simulink model "V2G_sim"  (R2021a)
settings: Solver=VariableStepAuto  StartTime=0  StopTime=tmax  FixedStep=sample_time  RelTol=1e-3  EnableMultiTasking=on
values from neighbouring files (symbols this model uses):
  Cap_car3_SC = 165    [V2G.m]
  grid_voltage = 230*sqrt(3)    [V2G.m]
  num_car1 = randi([1,50])    [V2G.m]
  num_car2 = randi([1,50])    [V2G.m]
  num_car3 = randi([1,50])    [V2G.m]
  pun = 40    [V2G.m]
  Qacc_MEAN = mean(Qacc_TOT, 1)    [V2G.m]
  sample_time = 0.0005    [V2G.m]
  V_car3_SC = 48    [V2G.m]
undefined symbols (not defined in the file or in its folder): Ion, Lithium
libraries: spsBreakerLib x8, spsCurrentMeasurementLib x8, spsVoltageMeasurementLib x8, spsMosfetLib x8, spsControlledCurrentSourceLib x4, spsSeriesRLCBranchLib x4, spsBatteryLib x3, simulink x2, spsSupercapacitorLib x1, spspowerguiLib x1
Description:
  | Copyright 2008-2016 The MathWorks, Inc.
settings Model: SimulationMode=accelerator  Creator=MathWorks  LastModifiedBy=rod
settings SolverCC: AlgebraicLoopSolver=TrustRegion
settings DataIOCC: FinalStateName=OperationPoint  InitialState=OperationPoint  LimitDataPoints=on  LoadInitialState=on  SaveFinalState=on  SaveOperatingPoint=on  SaveFormat=Array  SignalLoggingSaveFormat=ModelDataLogs  ReturnWorkspaceOutputs=off
settings OptimizationCC: BlockReduction=off  DefaultParameterBehavior=Inlined  BufferReuse=off  ExpressionDepthLimit=2147483647  EfficientMapNaN2IntZero=off  LifeSpan=inf
settings DebuggingCC: UnderspecifiedInitializationDetection=Classic  MergeDetectMultiDrivingBlocksExec=none  SolverPrmCheckMsg=warning  FcnCallInpInsideContextMsg=warning  UnconnectedInputMsg=none  UnconnectedOutputMsg=none  UnconnectedLineMsg=none  AllowSymbolicDim=off  StateNameClashWarn=warning  SFUnexpectedBacktrackingDiag=warning  SFNoUnconditionalDefaultTransitionDiag=warning  SFExecutionAtInitializationDiag=none  SFMachineParentedDataDiag=warning  ArithmeticOperatorsInVariantConditions=warning
settings HardwareCC: ProdBitPerPointer=32  ProdBitPerSizeT=32  ProdBitPerPtrDiffT=32  ProdLargestAtomicFloat=None  ProdIntDivRoundTo=Undefined  ProdEndianess=Unspecified  ProdWordSize=32  ProdHWDeviceType=32-bit Generic  TargetBitPerLong=64  TargetBitPerPointer=64  TargetBitPerSizeT=64  TargetBitPerPtrDiffT=64  TargetLongLongMode=on  TargetIntDivRoundTo=Zero  TargetEndianess=LittleEndian  TargetWordSize=64  TargetHWDeviceType=MATLAB Host  ProdEqTarget=off
settings ModelReferenceCC: PropagateSignalLabelsOutOfModel=off
settings SFSimCC: SimUseLocalCustomCode=off  CustomCodeUndefinedFunction=UseInterfaceOnly
settings RTWCC: SystemTargetFile=accel.tlc  TemplateMakefile=accel_default_tmf  RTWVerbose=off  RTWUseLocalCustomCode=off
settings CodeAppCC: MaxIdLength=128  StateflowObjectComments=on
settings STFCustomTargetCC: MATLABClassNameForMDSCustomization=Simulink.SoftwareTarget.TargetSpecificTriggerConfigurationBase  UseToolchainInfoCompliant=off  SystemTargetFile=accel.tlc
settings ConfigComp: CovMetricSettings=dw  CovSaveCumulativeToWorkspaceVar=on  CovSaveSingleToWorkspaceVar=on  CovExternalEMLEnable=off  CovSFcnEnable=off
settings SimscapeCC: SimscapeNormalizeSystem=off

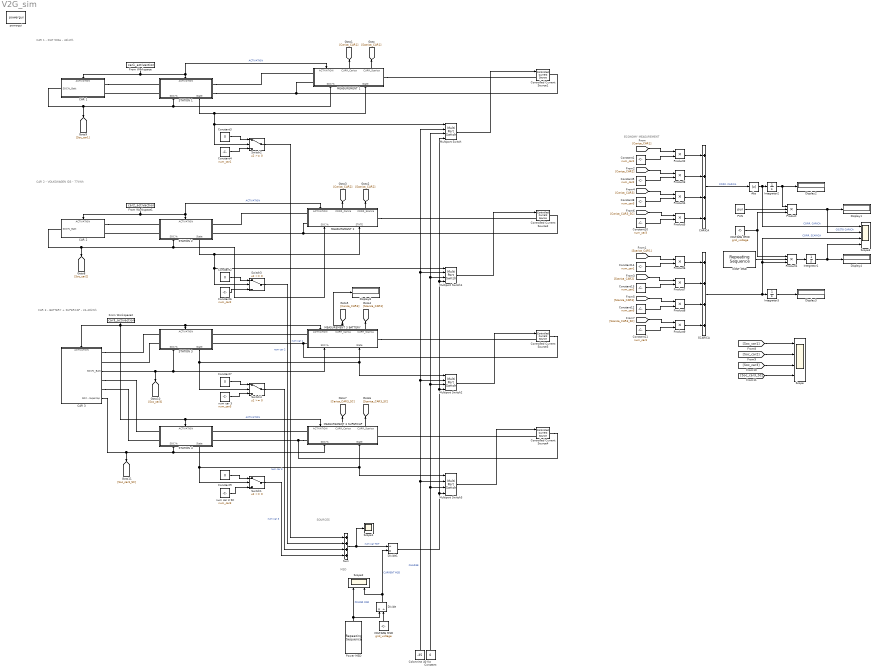
== system V2G_sim ==
  note: ECONOMY MEASUREMENT
  note: CAR 2 - VOLKSWAGEN ID3 - 77kWh
  note: SOURCES
  note: MSD
  note: CAR 1 - FIAT 500e - 42kWh
  note: CAR 3 - BATTERY + SUPERCAP - 24-40kWh
  Abs : Abs
  CAR 1 : Subsystem
      settings: PortSchema="{\"entries\":[{\"content\":{\"sides\":[{\"content\":{\"connectorIds\":[\"Out1\"]},\"type\":\"ConnectorPlacement.EquallySpacedRectSide\",\"uuid\":\"65240932-2f7c-4e6f-a11f-24cebb7f6932\"},{\"content\":{\"connectorIds\":[\"RConn1\",\"RConn2\"],\"side\":\"RIGHT\"},\"type\":\"ConnectorPlacement.EquallySpacedRectSide\",\"uuid\":\"fe08d712-a294-43ae-b558-1367f8f9eddb\"},{\"content\":{\"connectorIds\":[\"In1\"],\"side\":\"TOP\"},\"type\":\"ConnectorPlacement.EquallySpacedRectSide\",\"uuid\":\"eb8a317a-712b-4977-acdc-c1fc50b80e89\"},{\"content\":{\"connectorIds\":[],\"side\":\"BOTTOM\"},\"type\":\"ConnectorPlacement.EquallySpacedRectSide\",\"uuid\":\"4277e686-58a0-45df-b571-69968d3e8f8c\"}]},\"type\":\"ConnectorPlacement.EquallySpacedConnector\",\"uuid\":\"4b8ded93-b982-40b7-aa5b-c2f165d3142b\"}],\"packageUris\":[\"http://schema.mathworks.com/mf0/Connector/R2020b\"],\"version\":\"1.0\"}"
  CAR 2 : Subsystem
      settings: PortSchema="{\"entries\":[{\"content\":{\"sides\":[{\"content\":{\"connectorIds\":[\"Out1\"]},\"type\":\"ConnectorPlacement.EquallySpacedRectSide\",\"uuid\":\"65240932-2f7c-4e6f-a11f-24cebb7f6932\"},{\"content\":{\"connectorIds\":[\"RConn1\",\"RConn2\"],\"side\":\"RIGHT\"},\"type\":\"ConnectorPlacement.EquallySpacedRectSide\",\"uuid\":\"fe08d712-a294-43ae-b558-1367f8f9eddb\"},{\"content\":{\"connectorIds\":[\"In1\"],\"side\":\"TOP\"},\"type\":\"ConnectorPlacement.EquallySpacedRectSide\",\"uuid\":\"eb8a317a-712b-4977-acdc-c1fc50b80e89\"},{\"content\":{\"connectorIds\":[],\"side\":\"BOTTOM\"},\"type\":\"ConnectorPlacement.EquallySpacedRectSide\",\"uuid\":\"4277e686-58a0-45df-b571-69968d3e8f8c\"}]},\"type\":\"ConnectorPlacement.EquallySpacedConnector\",\"uuid\":\"4b8ded93-b982-40b7-aa5b-c2f165d3142b\"}],\"packageUris\":[\"http://schema.mathworks.com/mf0/Connector/R2020b\"],\"version\":\"1.0\"}"
  CAR 3 : Subsystem
      settings: PortSchema="{\"entries\":[{\"content\":{\"sides\":[{\"content\":{\"connectorIds\":[]},\"type\":\"ConnectorPlacement.EquallySpacedRectSide\",\"uuid\":\"65240932-2f7c-4e6f-a11f-24cebb7f6932\"},{\"content\":{\"connectorIds\":[\"RConn1\",\"RConn2\",\"Out1\",\"RConn3\",\"RConn4\",\"Out2\"],\"side\":\"RIGHT\"},\"type\":\"ConnectorPlacement.EquallySpacedRectSide\",\"uuid\":\"fe08d712-a294-43ae-b558-1367f8f9eddb\"},{\"content\":{\"connectorIds\":[\"In1\"],\"side\":\"TOP\"},\"type\":\"ConnectorPlacement.EquallySpacedRectSide\",\"uuid\":\"eb8a317a-712b-4977-acdc-c1fc50b80e89\"},{\"content\":{\"connectorIds\":[],\"side\":\"BOTTOM\"},\"type\":\"ConnectorPlacement.EquallySpacedRectSide\",\"uuid\":\"4277e686-58a0-45df-b571-69968d3e8f8c\"}]},\"type\":\"ConnectorPlacement.EquallySpacedConnector\",\"uuid\":\"4b8ded93-b982-40b7-aa5b-c2f165d3142b\"}],\"packageUris\":[\"http://schema.mathworks.com/mf0/Connector/R2020b\"],\"version\":\"1.0\"}"
  CARICA : Sum  Inputs=++++
  COST MSD : simulink/Sources/Repeating Sequence  rep_seq_t=time_var  rep_seq_y=Costo_MWh
  Colonnina 40 Kw : Constant  Value=-35
  Constant{,2..3,7,9} (5 alike) : Constant  Value=0
  Constant1 : Constant  Value=num_car1
  Constant{8,10..12} (4 alike) : Constant  Value=num_car3
  Constant13 : Constant  Value=num_car2
  Constant14 : Constant  Value=num_car1
  Constant4 : Constant  Value=num_car1
  Constant5 : Constant  Value=num_car2
  Constant6 : Constant  Value=num_car2
  Controlled Current Source{1..4} (4 alike) : spsControlledCurrentSourceLib/Controlled Current Source  Initialize=off  Source_Type=AC  Amplitude=0  Phase=0  Frequency=0  Measurements=None
  Display{1..4,8} (5 alike) : Display
  Divide : Product  Inputs=*/
  Divide1 : Product  Inputs=/*
  From Workspace : FromWorkspace  VariableName=car1_activaction  OutDataTypeStr=double  Interpolate=off  OutputAfterFinalValue=Holding final value
  From Workspace1 : FromWorkspace  VariableName=car2_activaction  OutDataTypeStr=double  Interpolate=off  OutputAfterFinalValue=Holding final value
  From Workspace2 : FromWorkspace  VariableName=car3_activaction  OutDataTypeStr=double  Interpolate=off  OutputAfterFinalValue=Holding final value
  Integrator1 : Integrator
  Integrator2 : Integrator
  Integrator3 : Integrator
  MEASUREMENT 1 : Subsystem
      settings: PortSchema="{\"entries\":[{\"content\":{\"sides\":[{\"content\":{\"connectorIds\":[\"LConn1\",\"LConn2\"]},\"type\":\"ConnectorPlacement.EquallySpacedRectSide\",\"uuid\":\"bd49ef22-917f-43a7-a189-1e95a09b9934\"},{\"content\":{\"connectorIds\":[\"RConn1\"],\"side\":\"RIGHT\"},\"type\":\"ConnectorPlacement.EquallySpacedRectSide\",\"uuid\":\"f047bc4d-f3d5-4ba6-b200-54db61941c53\"},{\"content\":{\"connectorIds\":[\"In1\",\"Out1\",\"Out2\"],\"side\":\"TOP\"},\"type\":\"ConnectorPlacement.EquallySpacedRectSide\",\"uuid\":\"9d09de71-fe9a-4093-9092-d12f300b0940\"},{\"content\":{\"connectorIds\":[\"In2\",\"In3\"],\"side\":\"BOTTOM\"},\"type\":\"ConnectorPlacement.EquallySpacedRectSide\",\"uuid\":\"f7496d22-be24-4c8d-8efb-c768b29ff46b\"}]},\"type\":\"ConnectorPlacement.EquallySpacedConnector\",\"uuid\":\"0e7a4336-45ad-4cd1-9eb0-8ed9ee74ee56\"}],\"packageUris\":[\"http://schema.mathworks.com/mf0/Connector/R2020b\"],\"version\":\"1.0\"}"
  MEASUREMENT 2 : Subsystem
      settings: PortSchema="{\"entries\":[{\"content\":{\"sides\":[{\"content\":{\"connectorIds\":[\"LConn1\",\"LConn2\"]},\"type\":\"ConnectorPlacement.EquallySpacedRectSide\",\"uuid\":\"bd49ef22-917f-43a7-a189-1e95a09b9934\"},{\"content\":{\"connectorIds\":[\"RConn1\"],\"side\":\"RIGHT\"},\"type\":\"ConnectorPlacement.EquallySpacedRectSide\",\"uuid\":\"f047bc4d-f3d5-4ba6-b200-54db61941c53\"},{\"content\":{\"connectorIds\":[\"In1\",\"Out1\",\"Out2\"],\"side\":\"TOP\"},\"type\":\"ConnectorPlacement.EquallySpacedRectSide\",\"uuid\":\"9d09de71-fe9a-4093-9092-d12f300b0940\"},{\"content\":{\"connectorIds\":[\"In2\",\"In3\"],\"side\":\"BOTTOM\"},\"type\":\"ConnectorPlacement.EquallySpacedRectSide\",\"uuid\":\"f7496d22-be24-4c8d-8efb-c768b29ff46b\"}]},\"type\":\"ConnectorPlacement.EquallySpacedConnector\",\"uuid\":\"0e7a4336-45ad-4cd1-9eb0-8ed9ee74ee56\"}],\"packageUris\":[\"http://schema.mathworks.com/mf0/Connector/R2020b\"],\"version\":\"1.0\"}"
  MEASUREMENT 3 BATTERY : Subsystem
      settings: PortSchema="{\"entries\":[{\"content\":{\"sides\":[{\"content\":{\"connectorIds\":[\"LConn1\",\"LConn2\"]},\"type\":\"ConnectorPlacement.EquallySpacedRectSide\",\"uuid\":\"bd49ef22-917f-43a7-a189-1e95a09b9934\"},{\"content\":{\"connectorIds\":[\"RConn1\"],\"side\":\"RIGHT\"},\"type\":\"ConnectorPlacement.EquallySpacedRectSide\",\"uuid\":\"f047bc4d-f3d5-4ba6-b200-54db61941c53\"},{\"content\":{\"connectorIds\":[\"In1\",\"Out1\",\"Out2\"],\"side\":\"TOP\"},\"type\":\"ConnectorPlacement.EquallySpacedRectSide\",\"uuid\":\"9d09de71-fe9a-4093-9092-d12f300b0940\"},{\"content\":{\"connectorIds\":[\"In2\",\"In3\"],\"side\":\"BOTTOM\"},\"type\":\"ConnectorPlacement.EquallySpacedRectSide\",\"uuid\":\"f7496d22-be24-4c8d-8efb-c768b29ff46b\"}]},\"type\":\"ConnectorPlacement.EquallySpacedConnector\",\"uuid\":\"0e7a4336-45ad-4cd1-9eb0-8ed9ee74ee56\"}],\"packageUris\":[\"http://schema.mathworks.com/mf0/Connector/R2020b\"],\"version\":\"1.0\"}"
  MEASUREMENT 3 SUPERCAP : Subsystem
      settings: PortSchema="{\"entries\":[{\"content\":{\"sides\":[{\"content\":{\"connectorIds\":[\"LConn1\",\"LConn2\"]},\"type\":\"ConnectorPlacement.EquallySpacedRectSide\",\"uuid\":\"bd49ef22-917f-43a7-a189-1e95a09b9934\"},{\"content\":{\"connectorIds\":[\"RConn1\"],\"side\":\"RIGHT\"},\"type\":\"ConnectorPlacement.EquallySpacedRectSide\",\"uuid\":\"f047bc4d-f3d5-4ba6-b200-54db61941c53\"},{\"content\":{\"connectorIds\":[\"In1\",\"Out1\",\"Out2\"],\"side\":\"TOP\"},\"type\":\"ConnectorPlacement.EquallySpacedRectSide\",\"uuid\":\"9d09de71-fe9a-4093-9092-d12f300b0940\"},{\"content\":{\"connectorIds\":[\"In2\",\"In3\"],\"side\":\"BOTTOM\"},\"type\":\"ConnectorPlacement.EquallySpacedRectSide\",\"uuid\":\"f7496d22-be24-4c8d-8efb-c768b29ff46b\"}]},\"type\":\"ConnectorPlacement.EquallySpacedConnector\",\"uuid\":\"0e7a4336-45ad-4cd1-9eb0-8ed9ee74ee56\"}],\"packageUris\":[\"http://schema.mathworks.com/mf0/Connector/R2020b\"],\"version\":\"1.0\"}"
  Multiport Switch{,1..3} (4 alike) : MultiPortSwitch  DataPortOrder=Specify indices  DataPortIndices={1,0,-1}  DiagnosticForDefault=None
  PUN : Constant  Value=pun
  Power MSD : simulink/Sources/Repeating Sequence  rep_seq_t=time_var  rep_seq_y=Qacc_MEAN*1e6
  Product : Product  Inputs=3
  Product1 : Product  Inputs=3
  Product{2..9} (8 alike) : Product
  SCARICA : Sum  Inputs=++++
  STATION 1 : Subsystem
      settings: PortSchema="{\"entries\":[{\"content\":{\"sides\":[{\"content\":{\"connectorIds\":[\"LConn1\",\"LConn2\"]},\"type\":\"ConnectorPlacement.EquallySpacedRectSide\",\"uuid\":\"f3913e7b-742e-4981-a29c-7d1eb9aabba7\"},{\"content\":{\"connectorIds\":[\"RConn1\",\"RConn2\"],\"side\":\"RIGHT\"},\"type\":\"ConnectorPlacement.EquallySpacedRectSide\",\"uuid\":\"c4f92920-f5e0-4664-9ed6-0c5e6a96934e\"},{\"content\":{\"connectorIds\":[\"In1\"],\"side\":\"TOP\"},\"type\":\"ConnectorPlacement.EquallySpacedRectSide\",\"uuid\":\"f98f0bbd-8b84-40b6-9fe0-725502f4315d\"},{\"content\":{\"connectorIds\":[\"In2\",\"Out1\"],\"side\":\"BOTTOM\"},\"type\":\"ConnectorPlacement.EquallySpacedRectSide\",\"uuid\":\"7bf24fc7-4b53-47e4-8856-ee368f4a74d7\"}]},\"type\":\"ConnectorPlacement.EquallySpacedConnector\",\"uuid\":\"8d316def-927b-4e3b-8675-f38de2cc490c\"}],\"packageUris\":[\"http://schema.mathworks.com/mf0/Connector/R2020b\"],\"version\":\"1.0\"}"
  STATION 2 : Subsystem
      settings: PortSchema="{\"entries\":[{\"content\":{\"sides\":[{\"content\":{\"connectorIds\":[\"LConn1\",\"LConn2\"]},\"type\":\"ConnectorPlacement.EquallySpacedRectSide\",\"uuid\":\"f3913e7b-742e-4981-a29c-7d1eb9aabba7\"},{\"content\":{\"connectorIds\":[\"RConn1\",\"RConn2\"],\"side\":\"RIGHT\"},\"type\":\"ConnectorPlacement.EquallySpacedRectSide\",\"uuid\":\"c4f92920-f5e0-4664-9ed6-0c5e6a96934e\"},{\"content\":{\"connectorIds\":[\"In1\"],\"side\":\"TOP\"},\"type\":\"ConnectorPlacement.EquallySpacedRectSide\",\"uuid\":\"f98f0bbd-8b84-40b6-9fe0-725502f4315d\"},{\"content\":{\"connectorIds\":[\"In2\",\"Out1\"],\"side\":\"BOTTOM\"},\"type\":\"ConnectorPlacement.EquallySpacedRectSide\",\"uuid\":\"7bf24fc7-4b53-47e4-8856-ee368f4a74d7\"}]},\"type\":\"ConnectorPlacement.EquallySpacedConnector\",\"uuid\":\"8d316def-927b-4e3b-8675-f38de2cc490c\"}],\"packageUris\":[\"http://schema.mathworks.com/mf0/Connector/R2020b\"],\"version\":\"1.0\"}"
  STATION 3 : Subsystem
      settings: PortSchema="{\"entries\":[{\"content\":{\"sides\":[{\"content\":{\"connectorIds\":[\"LConn1\",\"LConn2\"]},\"type\":\"ConnectorPlacement.EquallySpacedRectSide\",\"uuid\":\"f3913e7b-742e-4981-a29c-7d1eb9aabba7\"},{\"content\":{\"connectorIds\":[\"RConn1\",\"RConn2\"],\"side\":\"RIGHT\"},\"type\":\"ConnectorPlacement.EquallySpacedRectSide\",\"uuid\":\"c4f92920-f5e0-4664-9ed6-0c5e6a96934e\"},{\"content\":{\"connectorIds\":[\"In1\"],\"side\":\"TOP\"},\"type\":\"ConnectorPlacement.EquallySpacedRectSide\",\"uuid\":\"f98f0bbd-8b84-40b6-9fe0-725502f4315d\"},{\"content\":{\"connectorIds\":[\"In2\",\"Out1\"],\"side\":\"BOTTOM\"},\"type\":\"ConnectorPlacement.EquallySpacedRectSide\",\"uuid\":\"7bf24fc7-4b53-47e4-8856-ee368f4a74d7\"}]},\"type\":\"ConnectorPlacement.EquallySpacedConnector\",\"uuid\":\"8d316def-927b-4e3b-8675-f38de2cc490c\"}],\"packageUris\":[\"http://schema.mathworks.com/mf0/Connector/R2020b\"],\"version\":\"1.0\"}"
  STATION 4 : Subsystem
      settings: PortSchema="{\"entries\":[{\"content\":{\"sides\":[{\"content\":{\"connectorIds\":[\"LConn1\",\"LConn2\"]},\"type\":\"ConnectorPlacement.EquallySpacedRectSide\",\"uuid\":\"f3913e7b-742e-4981-a29c-7d1eb9aabba7\"},{\"content\":{\"connectorIds\":[\"RConn1\",\"RConn2\"],\"side\":\"RIGHT\"},\"type\":\"ConnectorPlacement.EquallySpacedRectSide\",\"uuid\":\"c4f92920-f5e0-4664-9ed6-0c5e6a96934e\"},{\"content\":{\"connectorIds\":[\"In1\"],\"side\":\"TOP\"},\"type\":\"ConnectorPlacement.EquallySpacedRectSide\",\"uuid\":\"f98f0bbd-8b84-40b6-9fe0-725502f4315d\"},{\"content\":{\"connectorIds\":[\"In2\",\"Out1\"],\"side\":\"BOTTOM\"},\"type\":\"ConnectorPlacement.EquallySpacedRectSide\",\"uuid\":\"7bf24fc7-4b53-47e4-8856-ee368f4a74d7\"}]},\"type\":\"ConnectorPlacement.EquallySpacedConnector\",\"uuid\":\"8d316def-927b-4e3b-8675-f38de2cc490c\"}],\"packageUris\":[\"http://schema.mathworks.com/mf0/Connector/R2020b\"],\"version\":\"1.0\"}"
  Scope : Scope  NumInputPorts=4
  Scope1 : Scope
  Scope2 : Scope  NumInputPorts=2
  Scope3 : Scope  NumInputPorts=4
  Sum : Sum  Inputs=++++
  Switch{1..4} (4 alike) : Switch
  VOLTAGE GRID : Constant  Value=grid_voltage
  VOLTAGE MSD : Constant  Value=grid_voltage
  num car 3 : Constant  Value=num_car3
  num car 3 SC : Constant  Value=num_car3
  powergui : spspowerguiLib/powergui  Priority=1  SimulationMode=Discrete  SampleTime=sample_time  frequency=60  Iterations=50  frequencyindice=0  Pbase=100e6  ErrMax=1e-4  UnitsV=kV  UnitsW=MW  buscounter=0  FunctionMessages=off  echomessages=off  EnableUseOfTLC=off  CurrentSourceSwitches=off  DisableSnubberDevices=off  DisableRonSwitches=off  DisableVfSwitches=off  DisplayEquations=off  AutomaticDiscreteSolvers=off  SolverType=Tustin/Backward Euler (TBE)  Interpol=off  ExternalGateDelay=off  methode=off  Ts=0  x0status=blocks  SPID=off  SwTol=0  HookPort=off  NonlinearTolerance=1e-2  nMaxIteration=100  ContinueOnMaxIteration=off  RestoreLinks=warning  ResistiveCurrentMeasurement=off  Frange=[0:1:1000]  Ylog=on  Xlog=on  ShowGrid=on  save=on  variable=ZDa  structure=donnee  ZoomFFT=off  StartTime=0.0  cycles=1  DisplayStyle=1  fundamental=60  FreqAxis=off  MaxFrequency=1000  frequencyindicesteady=10  RmsSteady=1  display=off
  wires:
  Power MSD/1 -> Divide/1, Scope2/1  "POWER MSD"
  VOLTAGE MSD/1 -> Divide/2
  Colonnina 40 Kw/1 -> Multiport Switch1/2, Multiport Switch/2, Multiport Switch2/2, Multiport Switch3/2  "CHARGE"
  Integrator2/1 -> Display2/1, Product/1
  Divide/1 -> Divide1/2, Scope2/2  "CURRENT MSD"
  CARICA/1 -> Abs/1  "CORR. CARICA"
  STATION 1/1(State) -> MEASUREMENT 1/3(State), Switch2/2, Multiport Switch/1
  Divide1/1 -> Multiport Switch3/4, Multiport Switch/4, Multiport Switch1/4, Multiport Switch2/4
  From Workspace/1 -> CAR 1/1(ACTIVATION), STATION 1/1(ACTIVATION), MEASUREMENT 1/1(ACTIVATION)  "ACTIVATION"
  CAR 1/1(SOC%_Batt) -> [Soc_car1], MEASUREMENT 1/2(SOC %), STATION 1/2(SOC %)
  Constant3/1 -> Switch2/1
  Constant4/1 -> Switch2/3
  Switch2/1 -> Sum/1  "num car 1"
  STATION 2/1(State) -> MEASUREMENT 2/3(STATE), Switch3/2, Multiport Switch1/1
  From Workspace1/1 -> CAR 2/1(ACTIVATION), STATION 2/1(ACTIVATION), MEASUREMENT 2/1(ACTIVATION)  "ACTIVATION"
  Constant6/1 -> Switch3/3
  Constant2/1 -> Switch3/1
  CAR 2/1(SOC%_Batt) -> [Soc_car2], MEASUREMENT 2/2(SOC %), STATION 2/2(SOC %)
  Switch3/1 -> Sum/2  "num car 2"
  From Workspace2/1 -> MEASUREMENT 3 SUPERCAP/1(ACTIVATION), STATION 4/1(ACTIVATION), CAR 3/1(ACTIVATION), MEASUREMENT 3 BATTERY/1(ACTIVATION), STATION 3/1(ACTIVATION)  "ACTIVATION"
  STATION 3/1(State) -> Multiport Switch2/1, MEASUREMENT 3 BATTERY/3(State), Switch4/2
  CAR 3/1(SOC%_Batt) -> [Soc_car3], MEASUREMENT 3 BATTERY/2(SOC %), STATION 3/2(SOC %)
  Switch4/1 -> Sum/3  "num car 3"
  Multiport Switch1/1 -> Controlled Current Source2/1
  Multiport Switch/1 -> Controlled Current Source1/1
  Constant/1 -> Multiport Switch1/3, Multiport Switch/3, Multiport Switch2/3, Multiport Switch3/3
  MEASUREMENT 1/1(CURR_Carica) -> [Carica_CAR1]
  MEASUREMENT 1/2(CURR_Scarica) -> [Scarica_CAR1]
  PUN/1 -> Product/2
  COST MSD/1 -> Product1/2
  MEASUREMENT 2/2(CORR_Scarica) -> [Scarica_CAR2]
  MEASUREMENT 2/1(CORR_Carica) -> [Carica_CAR2]
  MEASUREMENT 3 BATTERY/1(CURR_Carica) -> Display8/1, [Carica_CAR3]
  MEASUREMENT 3 BATTERY/2(CURR_Scarica) -> [Scarica_CAR3]
  CAR 3/2(SOC%_Supercap) -> MEASUREMENT 3 SUPERCAP/2(SOC %), STATION 4/2(SOC %), [Soc_car3_SC]
  Constant7/1 -> Switch4/1
  Multiport Switch2/1 -> Controlled Current Source3/1
  [Soc_car1] -> Scope/1
  [Soc_car2] -> Scope/2
  [Soc_car3] -> Scope/3
  [Soc_car3_SC] -> Scope/4
  Abs/1 -> Scope3/1, Integrator2/1  "CORR. CARICA"
  VOLTAGE GRID/1 -> Product/3, Product1/1
  SCARICA/1 -> Product1/3, Scope3/3, Integrator3/1  "CORR. SCARICA"
  Integrator3/1 -> Display3/1
  Product1/1 -> Integrator1/1
  Product/1 -> Display1/1, Scope3/2  "COSTO CARICA"
  Multiport Switch3/1 -> Controlled Current Source4/1
  MEASUREMENT 3 SUPERCAP/1(CURR_Carica) -> [Carica_CAR3_SC]
  MEASUREMENT 3 SUPERCAP/2(CURR_Scarica) -> [Scarica_CAR3_SC]
  STATION 4/1(State) -> Switch1/2, Multiport Switch3/1, MEASUREMENT 3 SUPERCAP/3(State)
  Sum/1 -> Divide1/1, Scope1/1  "num car TOT"
  Constant9/1 -> Switch1/1
  num car 3 SC/1 -> Switch1/3
  Switch1/1 -> Sum/4  "num car 3"
  num car 3/1 -> Switch4/3
  Product2/1 -> CARICA/1
  [Carica_CAR1] -> Product2/1
  Constant1/1 -> Product2/2
  Product3/1 -> CARICA/2
  Product4/1 -> CARICA/3
  Product5/1 -> CARICA/4
  [Carica_CAR2] -> Product3/1
  Constant5/1 -> Product3/2
  Constant8/1 -> Product4/2
  [Carica_CAR3] -> Product4/1
  [Carica_CAR3_SC] -> Product5/1
  Constant10/1 -> Product5/2
  Product6/1 -> SCARICA/1
  Product7/1 -> SCARICA/2
  Product8/1 -> SCARICA/3
  Product9/1 -> SCARICA/4
  [Scarica_CAR1] -> Product6/1
  Constant14/1 -> Product6/2
  Constant11/1 -> Product9/2
  [Scarica_CAR3_SC] -> Product9/1
  Constant12/1 -> Product8/2
  [Scarica_CAR3] -> Product8/1
  [Scarica_CAR2] -> Product7/1
  Constant13/1 -> Product7/2
  Integrator1/1 -> Scope3/4, Display4/1
  connections:
  STATION 1/RConn2 -- Controlled Current Source1/RConn1 -- MEASUREMENT 1/LConn2
  CAR 1/RConn1 -- STATION 1/LConn1
  STATION 1/LConn2 -- CAR 1/RConn2
  CAR 2/RConn1 -- STATION 2/LConn1
  MEASUREMENT 2/LConn2 -- Controlled Current Source2/RConn1 -- STATION 2/RConn2
  STATION 2/LConn2 -- CAR 2/RConn2
  STATION 3/LConn2 -- CAR 3/RConn2
  CAR 3/RConn1 -- STATION 3/LConn1
  STATION 1/RConn1 -- MEASUREMENT 1/LConn1
  MEASUREMENT 1/RConn1 -- Controlled Current Source1/LConn1
  MEASUREMENT 2/LConn1 -- STATION 2/RConn1
  MEASUREMENT 2/RConn1 -- Controlled Current Source2/LConn1
  MEASUREMENT 3 BATTERY/RConn1 -- Controlled Current Source3/LConn1
  MEASUREMENT 3 BATTERY/LConn1 -- STATION 3/RConn1
  MEASUREMENT 3 BATTERY/LConn2 -- Controlled Current Source3/RConn1 -- STATION 3/RConn2
  MEASUREMENT 3 SUPERCAP/LConn1 -- STATION 4/RConn1
  MEASUREMENT 3 SUPERCAP/LConn2 -- STATION 4/RConn2 -- Controlled Current Source4/RConn1
  CAR 3/RConn3 -- STATION 4/LConn1
  CAR 3/RConn4 -- STATION 4/LConn2
  Controlled Current Source4/LConn1 -- MEASUREMENT 3 SUPERCAP/RConn1

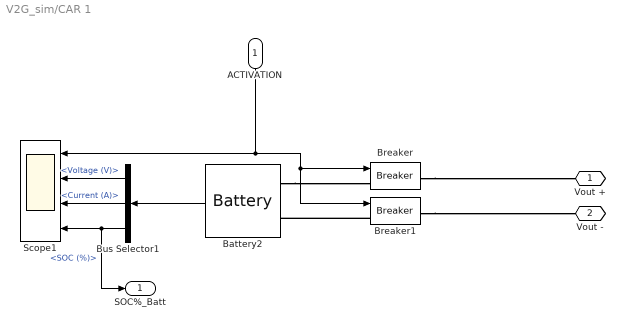
== system V2G_sim/CAR 1 ==
  ACTIVATION : Inport
  Battery2 : spsBatteryLib/Battery  BatType=Lithium-Ion  ShowTempParam=off  ThermalPreset=no  ShowAgeParam=off  NomV=Vbn_car1  NomQ=Ahn_car1  SOC=Soc0_car1  Batt_Tr=30  PresetModel=on  MaxQ=120  MinV=262.5  FullV=407.3955  Dis_rate=52.1739  R=0.029167  Normal_OP=108.5217  expZone="[378.135      5.895652]"  current=[6.5 13 32.5]  Units=Time  Tci=20  NomT=25  T2=0  MaxQ2=2.208  FullV2=3.45  Normal_OP2=2.8  expZone2="[3.22        0.23]"  Rca=0.6  ti=1000  Dp=0  Neq0=0  Tsim=1e6  Ta1=25  Qeol=5.4*0.9  Reol=0.013333*1.2  Char_age=[2.3478, 3]  Dis_age=[2.3478, 10]  N1=1500  N2=10500  N3=1000  N4=1400  Ta2=45  N5=950
  Breaker : spsBreakerLib/Breaker  InitialState=0  SwitchingTimes="[1/60  5/60]"  External=on  BreakerResistance=0.01  SnubberResistance=1e12  SnubberCapacitance=inf  Measurements=None  MoreParameters=on  NoBreakLoop=off
      settings: SourceProductBaseCode=PS
  Breaker1 : spsBreakerLib/Breaker  InitialState=0  SwitchingTimes="[1/60  5/60]"  External=on  BreakerResistance=0.01  SnubberResistance=1e12  SnubberCapacitance=inf  Measurements=None  MoreParameters=on  NoBreakLoop=off
      settings: SourceProductBaseCode=PS
  Bus Selector1 : BusSelector  OutputSignals=Voltage (V),Current (A),SOC (%)
  Scope1 : Scope  NumInputPorts=4
  Vout + : PMIOPort  Side=Right
  Vout - : PMIOPort  Port=2  Side=Right
  SOC%_Batt : Outport
  wires:
  Bus Selector1/2 -> Scope1/3  "<Current (A)>"
  Bus Selector1/3 -> SOC%_Batt/1, Scope1/4  "<SOC (%)>"
  Battery2/1 -> Bus Selector1/1
  Bus Selector1/1 -> Scope1/2  "<Voltage (V)>"
  ACTIVATION/1 -> Breaker/1, Breaker1/1, Scope1/1
  connections:
  Breaker1/RConn1 -- Vout -/RConn1
  Breaker1/LConn1 -- Battery2/LConn2
  Battery2/LConn1 -- Breaker/LConn1
  Breaker/RConn1 -- Vout +/RConn1

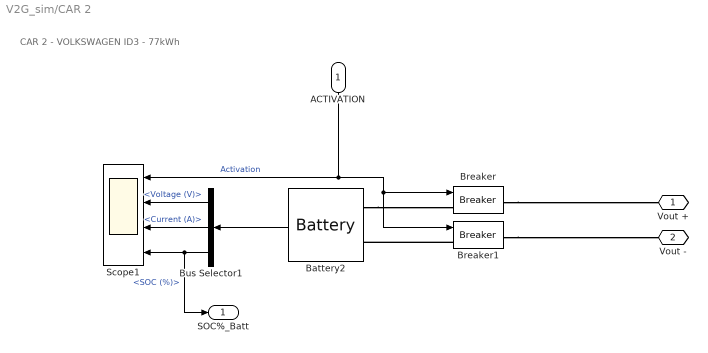
== system V2G_sim/CAR 2 ==
  note: CAR 2 - VOLKSWAGEN ID3 - 77kWh
  ACTIVATION : Inport
  Battery2 : spsBatteryLib/Battery  BatType=Lithium-Ion  ShowTempParam=off  ThermalPreset=no  ShowAgeParam=off  NomV=Vbn_car2  NomQ=Ahn_car2  SOC=Soc0_car2  Batt_Tr=30  PresetModel=on  MaxQ=185  MinV=306  FullV=474.9068  Dis_rate=80.4348  R=0.022054  Normal_OP=167.3043  expZone="[440.7974       9.08913]"  current=[6.5 13 32.5]  Units=Time  Tci=20  NomT=25  T2=0  MaxQ2=2.208  FullV2=3.45  Normal_OP2=2.8  expZone2="[3.22        0.23]"  Rca=0.6  ti=1000  Dp=0  Neq0=0  Tsim=1e6  Ta1=25  Qeol=5.4*0.9  Reol=0.013333*1.2  Char_age=[2.3478, 3]  Dis_age=[2.3478, 10]  N1=1500  N2=10500  N3=1000  N4=1400  Ta2=45  N5=950
  Breaker : spsBreakerLib/Breaker  InitialState=0  SwitchingTimes="[1/60  5/60]"  External=on  BreakerResistance=0.01  SnubberResistance=1e12  SnubberCapacitance=inf  Measurements=None  MoreParameters=on  NoBreakLoop=off
      settings: SourceProductBaseCode=PS
  Breaker1 : spsBreakerLib/Breaker  InitialState=0  SwitchingTimes="[1/60  5/60]"  External=on  BreakerResistance=0.01  SnubberResistance=1e12  SnubberCapacitance=inf  Measurements=None  MoreParameters=on  NoBreakLoop=off
      settings: SourceProductBaseCode=PS
  Bus Selector1 : BusSelector  OutputSignals=Voltage (V),Current (A),SOC (%)
  Scope1 : Scope  NumInputPorts=4
  Vout + : PMIOPort  Side=Right
  Vout - : PMIOPort  Port=2  Side=Right
  SOC%_Batt : Outport
  wires:
  Bus Selector1/2 -> Scope1/3  "<Current (A)>"
  Bus Selector1/3 -> SOC%_Batt/1, Scope1/4  "<SOC (%)>"
  Battery2/1 -> Bus Selector1/1
  Bus Selector1/1 -> Scope1/2  "<Voltage (V)>"
  ACTIVATION/1 -> Breaker/1, Breaker1/1, Scope1/1  "Activation"
  connections:
  Breaker1/RConn1 -- Vout -/RConn1
  Breaker1/LConn1 -- Battery2/LConn2
  Battery2/LConn1 -- Breaker/LConn1
  Breaker/RConn1 -- Vout +/RConn1

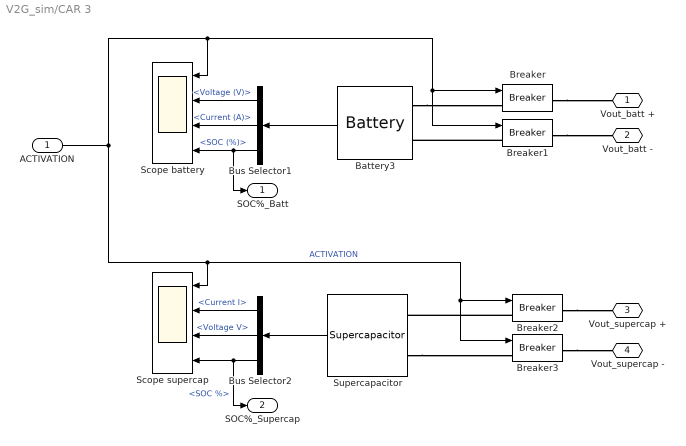
== system V2G_sim/CAR 3 ==
  ACTIVATION : Inport
  Battery3 : spsBatteryLib/Battery  BatType=Lithium-Ion  ShowTempParam=off  ThermalPreset=no  ShowAgeParam=off  NomV=Vbn_car3  NomQ=Ahn_car3  SOC=Soc0_car3  Batt_Tr=30  PresetModel=on  MaxQ=66  MinV=273  FullV=423.6913  Dis_rate=28.6957  R=0.055152  Normal_OP=59.687  expZone="[393.2605      3.242609]"  current=[6.5 13 32.5]  Units=Time  Tci=20  NomT=25  T2=0  MaxQ2=2.208  FullV2=3.45  Normal_OP2=2.8  expZone2="[3.22        0.23]"  Rca=0.6  ti=1000  Dp=0  Neq0=0  Tsim=1e6  Ta1=25  Qeol=5.4*0.9  Reol=0.013333*1.2  Char_age=[2.3478, 3]  Dis_age=[2.3478, 10]  N1=1500  N2=10500  N3=1000  N4=1400  Ta2=45  N5=950
  Breaker{,1..3} (4 alike) : spsBreakerLib/Breaker  InitialState=0  SwitchingTimes="[1/60  5/60]"  External=on  BreakerResistance=0.01  SnubberResistance=1e12  SnubberCapacitance=inf  Measurements=None  MoreParameters=on  NoBreakLoop=off
      settings: SourceProductBaseCode=PS
  Bus Selector1 : BusSelector  OutputSignals=Voltage (V),Current (A),SOC (%)
  Bus Selector2 : BusSelector  OutputSignals=Current I,Voltage V,SOC %
  Scope battery : Scope  NumInputPorts=4
  Scope supercap : Scope  NumInputPorts=4
  Supercapacitor : spsSupercapacitorLib/Supercapacitor  C=Cap_car3_SC  Rdc=ESR_car3_SC  Voltage=V_car3_SC  Ns=Nseries_car3_SC  Np=Nparallel_car3_SC  Vinit=Soc0_car3_SC  Temp=25  PresetModel=on  EstParam=off  Nc=1  r=1e-9  epsilon=6.0208e-10  Ich=10  Vstern="[0.161  2.7  7.8]"  Self_dis=off  Ioc=10  Vself="[48  47.8  47.06  44.65]"  demandeplot=off  I="[10  20 100  500]"  Units=sec  Vmax=0  If=0  deltaV=0  alpha=0  sec=0
      settings: SourceProductBaseCode=PS
  Vout_batt + : PMIOPort  Side=Right
  Vout_batt - : PMIOPort  Port=2  Side=Right
  Vout_supercap + : PMIOPort  Port=3  Side=Right
  Vout_supercap - : PMIOPort  Port=4  Side=Right
  SOC%_Batt : Outport
  SOC%_Supercap : Outport  Port=2
  wires:
  Bus Selector1/2 -> Scope battery/3  "<Current (A)>"
  Bus Selector1/3 -> SOC%_Batt/1, Scope battery/4  "<SOC (%)>"
  Battery3/1 -> Bus Selector1/1
  Bus Selector1/1 -> Scope battery/2  "<Voltage (V)>"
  ACTIVATION/1 -> Breaker/1, Breaker1/1, Scope battery/1, Scope supercap/1, Breaker3/1, Breaker2/1  "ACTIVATION"
  Bus Selector2/1 -> Scope supercap/2  "<Current I>"
  Bus Selector2/3 -> Scope supercap/4, SOC%_Supercap/1  "<SOC %>"
  Bus Selector2/2 -> Scope supercap/3  "<Voltage V>"
  Supercapacitor/1 -> Bus Selector2/1
  connections:
  Breaker1/RConn1 -- Vout_batt -/RConn1
  Breaker1/LConn1 -- Battery3/LConn2
  Battery3/LConn1 -- Breaker/LConn1
  Breaker/RConn1 -- Vout_batt +/RConn1
  Breaker2/RConn1 -- Vout_supercap +/RConn1
  Breaker3/RConn1 -- Vout_supercap -/RConn1
  Breaker2/LConn1 -- Supercapacitor/LConn1
  Supercapacitor/LConn2 -- Breaker3/LConn1

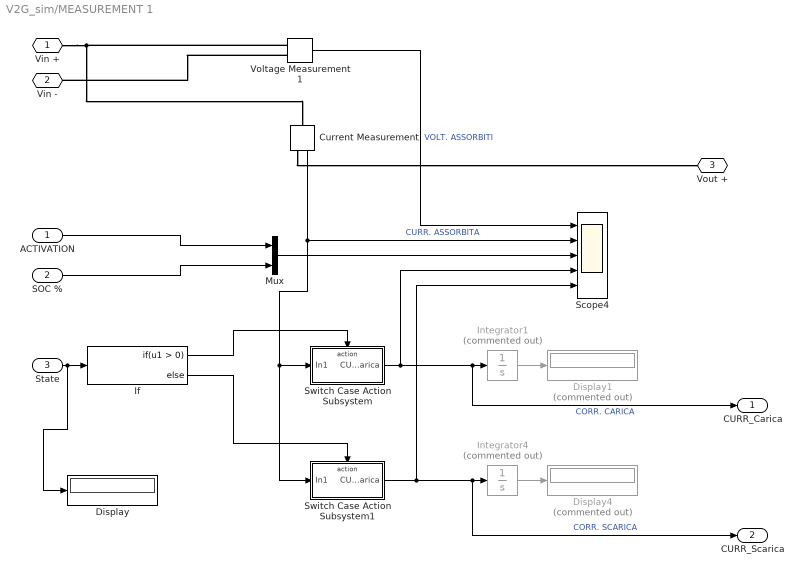
== system V2G_sim/MEASUREMENT 1 ==
  ACTIVATION : Inport
  SOC % : Inport  Port=2
  State : Inport  Port=3
  Current Measurement : spsCurrentMeasurementLib/Current Measurement  PhasorSimulation=off  OutputType=Complex  PSBequivalent=0
  Display : Display
  Display1 : Display  Commented=on
  Display4 : Display  Commented=on
  If : If
  Integrator1 : Integrator  Commented=on
  Integrator4 : Integrator  Commented=on
  Mux : Mux  Inputs=2
  Scope4 : Scope  NumInputPorts=5
  Switch Case Action Subsystem : Subsystem  TreatAsAtomicUnit=on
  Switch Case Action Subsystem1 : Subsystem  TreatAsAtomicUnit=on
  Voltage Measurement1 : spsVoltageMeasurementLib/Voltage Measurement  PhasorSimulation=off  OutputType=Complex  PSBequivalent=0
  Vin + : PMIOPort  Side=Left
  Vin - : PMIOPort  Port=2  Side=Left
  Vout + : PMIOPort  Port=3  Side=Right
  CURR_Carica : Outport
  CURR_Scarica : Outport  Port=2
  wires:
  Integrator4/1 -> Display4/1
  ACTIVATION/1 -> Mux/1
  Integrator1/1 -> Display1/1
  Switch Case Action Subsystem/1(CURR_Carica) -> Scope4/4, CURR_Carica/1, Integrator1/1  "CORR. CARICA"
  SOC %/1 -> Mux/2
  Voltage Measurement1/1 -> Scope4/1  "VOLT. ASSORBITI"
  Mux/1 -> Scope4/3
  Current Measurement/1 -> Switch Case Action Subsystem1/1(In1), Switch Case Action Subsystem/1(In1), Scope4/2  "CURR. ASSORBITA"
  Switch Case Action Subsystem1/1(CURR_Scarica) -> Scope4/5, CURR_Scarica/1, Integrator4/1  "CORR. SCARICA"
  State/1 -> Display/1, If/1
  If/1 -> Switch Case Action Subsystem/Action
  If/2 -> Switch Case Action Subsystem1/Action
  connections:
  Voltage Measurement1/LConn2 -- Vin -/RConn1
  Current Measurement/RConn1 -- Vout +/RConn1
  Voltage Measurement1/LConn1 -- Vin +/RConn1 -- Current Measurement/LConn1

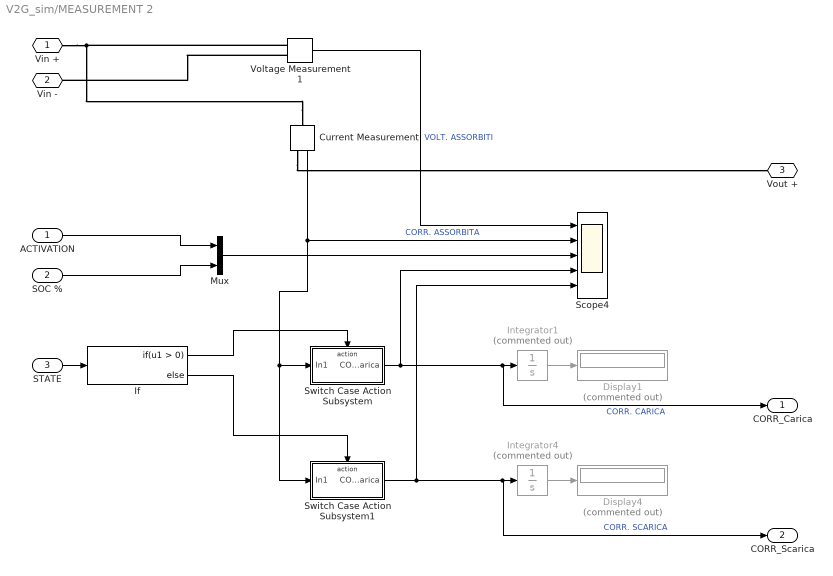
== system V2G_sim/MEASUREMENT 2 ==
  ACTIVATION : Inport
  SOC % : Inport  Port=2
  STATE : Inport  Port=3
  Current Measurement : spsCurrentMeasurementLib/Current Measurement  PhasorSimulation=off  OutputType=Complex  PSBequivalent=0
  Display1 : Display  Commented=on
  Display4 : Display  Commented=on
  If : If
  Integrator1 : Integrator  Commented=on
  Integrator4 : Integrator  Commented=on
  Mux : Mux  Inputs=2
  Scope4 : Scope  NumInputPorts=5
  Switch Case Action Subsystem : Subsystem  TreatAsAtomicUnit=on
  Switch Case Action Subsystem1 : Subsystem  TreatAsAtomicUnit=on
  Voltage Measurement1 : spsVoltageMeasurementLib/Voltage Measurement  PhasorSimulation=off  OutputType=Complex  PSBequivalent=0
  Vin + : PMIOPort  Side=Left
  Vin - : PMIOPort  Port=2  Side=Left
  Vout + : PMIOPort  Port=3  Side=Right
  CORR_Carica : Outport
  CORR_Scarica : Outport  Port=2
  wires:
  If/2 -> Switch Case Action Subsystem1/Action
  If/1 -> Switch Case Action Subsystem/Action
  STATE/1 -> If/1
  Switch Case Action Subsystem1/1(CORR_Scarica) -> Integrator4/1, CORR_Scarica/1, Scope4/5  "CORR. SCARICA"
  Current Measurement/1 -> Scope4/2, Switch Case Action Subsystem/1(In1), Switch Case Action Subsystem1/1(In1)  "CORR. ASSORBITA"
  Mux/1 -> Scope4/3
  Voltage Measurement1/1 -> Scope4/1  "VOLT. ASSORBITI"
  SOC %/1 -> Mux/2
  Switch Case Action Subsystem/1(CORR_Carica) -> Integrator1/1, CORR_Carica/1, Scope4/4  "CORR. CARICA"
  Integrator1/1 -> Display1/1
  ACTIVATION/1 -> Mux/1
  Integrator4/1 -> Display4/1
  connections:
  Current Measurement/LConn1 -- Vin +/RConn1 -- Voltage Measurement1/LConn1
  Current Measurement/RConn1 -- Vout +/RConn1
  Voltage Measurement1/LConn2 -- Vin -/RConn1

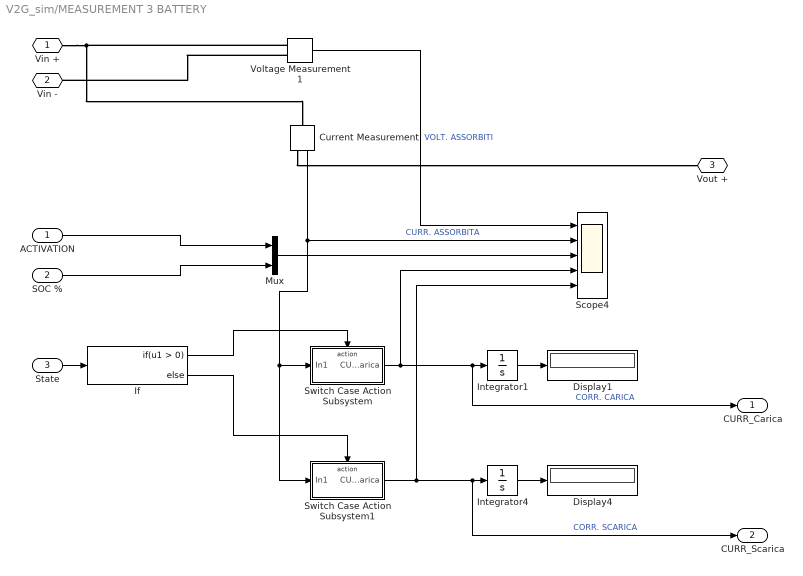
== system V2G_sim/MEASUREMENT 3 BATTERY ==
  ACTIVATION : Inport
  SOC % : Inport  Port=2
  State : Inport  Port=3
  Current Measurement : spsCurrentMeasurementLib/Current Measurement  PhasorSimulation=off  OutputType=Complex  PSBequivalent=0
  Display1 : Display
  Display4 : Display
  If : If
  Integrator1 : Integrator
  Integrator4 : Integrator
  Mux : Mux  Inputs=2
  Scope4 : Scope  NumInputPorts=5
  Switch Case Action Subsystem : Subsystem  TreatAsAtomicUnit=on
  Switch Case Action Subsystem1 : Subsystem  TreatAsAtomicUnit=on
  Voltage Measurement1 : spsVoltageMeasurementLib/Voltage Measurement  PhasorSimulation=off  OutputType=Complex  PSBequivalent=0
  Vin + : PMIOPort  Side=Left
  Vin - : PMIOPort  Port=2  Side=Left
  Vout + : PMIOPort  Port=3  Side=Right
  CURR_Carica : Outport
  CURR_Scarica : Outport  Port=2
  wires:
  Integrator4/1 -> Display4/1
  ACTIVATION/1 -> Mux/1
  Integrator1/1 -> Display1/1
  Switch Case Action Subsystem/1(CURR_Carica) -> Scope4/4, CURR_Carica/1, Integrator1/1  "CORR. CARICA"
  SOC %/1 -> Mux/2
  Voltage Measurement1/1 -> Scope4/1  "VOLT. ASSORBITI"
  Mux/1 -> Scope4/3
  Current Measurement/1 -> Switch Case Action Subsystem1/1(In1), Switch Case Action Subsystem/1(In1), Scope4/2  "CURR. ASSORBITA"
  Switch Case Action Subsystem1/1(CURR_Scarica) -> Scope4/5, CURR_Scarica/1, Integrator4/1  "CORR. SCARICA"
  State/1 -> If/1
  If/1 -> Switch Case Action Subsystem/Action
  If/2 -> Switch Case Action Subsystem1/Action
  connections:
  Voltage Measurement1/LConn2 -- Vin -/RConn1
  Current Measurement/RConn1 -- Vout +/RConn1
  Voltage Measurement1/LConn1 -- Vin +/RConn1 -- Current Measurement/LConn1

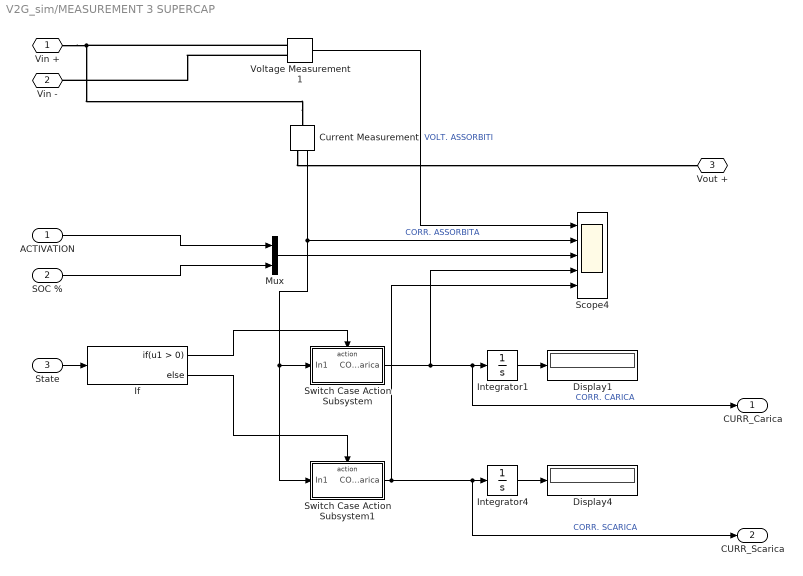
== system V2G_sim/MEASUREMENT 3 SUPERCAP ==
  ACTIVATION : Inport
  SOC % : Inport  Port=2
  State : Inport  Port=3
  Current Measurement : spsCurrentMeasurementLib/Current Measurement  PhasorSimulation=off  OutputType=Complex  PSBequivalent=0
  Display1 : Display
  Display4 : Display
  If : If
  Integrator1 : Integrator
  Integrator4 : Integrator
  Mux : Mux  Inputs=2
  Scope4 : Scope  NumInputPorts=5
  Switch Case Action Subsystem : Subsystem  TreatAsAtomicUnit=on
  Switch Case Action Subsystem1 : Subsystem  TreatAsAtomicUnit=on
  Voltage Measurement1 : spsVoltageMeasurementLib/Voltage Measurement  PhasorSimulation=off  OutputType=Complex  PSBequivalent=0
  Vin + : PMIOPort  Side=Left
  Vin - : PMIOPort  Port=2  Side=Left
  Vout + : PMIOPort  Port=3  Side=Right
  CURR_Carica : Outport
  CURR_Scarica : Outport  Port=2
  wires:
  If/2 -> Switch Case Action Subsystem1/Action
  If/1 -> Switch Case Action Subsystem/Action
  State/1 -> If/1
  Switch Case Action Subsystem1/1(CORR_Scarica) -> Integrator4/1, CURR_Scarica/1, Scope4/5  "CORR. SCARICA"
  Current Measurement/1 -> Scope4/2, Switch Case Action Subsystem/1(In1), Switch Case Action Subsystem1/1(In1)  "CORR. ASSORBITA"
  Mux/1 -> Scope4/3
  Voltage Measurement1/1 -> Scope4/1  "VOLT. ASSORBITI"
  SOC %/1 -> Mux/2
  Switch Case Action Subsystem/1(CORR_Carica) -> Integrator1/1, CURR_Carica/1, Scope4/4  "CORR. CARICA"
  Integrator1/1 -> Display1/1
  ACTIVATION/1 -> Mux/1
  Integrator4/1 -> Display4/1
  connections:
  Current Measurement/LConn1 -- Vin +/RConn1 -- Voltage Measurement1/LConn1
  Current Measurement/RConn1 -- Vout +/RConn1
  Voltage Measurement1/LConn2 -- Vin -/RConn1

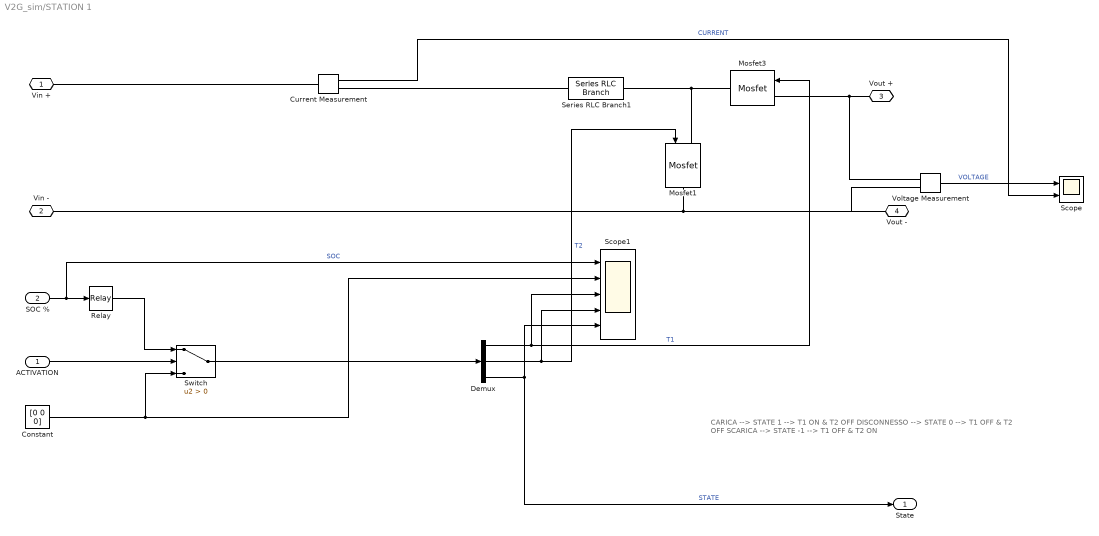
== system V2G_sim/STATION 1 ==
  note: CARICA --> STATE 1 --> T1 ON & T2 OFF
      | DISCONNESSO --> STATE 0 --> T1 OFF & T2 OFF
      | SCARICA --> STATE -1 --> T1 OFF & T2 ON
  ACTIVATION : Inport
  SOC % : Inport  Port=2
  Constant : Constant  Value=[0 0 0]
  Current Measurement : spsCurrentMeasurementLib/Current Measurement  PhasorSimulation=off  OutputType=Complex  PSBequivalent=0
  Demux : Demux  Outputs=3
  Mosfet1 : spsMosfetLib/Mosfet  Ron=0.1  Lon=0  Rd=0.01  Vfd=0  IC=0  Rs=1e5  Cs=inf  Measurements=off
  Mosfet3 : spsMosfetLib/Mosfet  Ron=0.1  Lon=0  Rd=0.01  Vfd=0  IC=0  Rs=1e5  Cs=inf  Measurements=off
  Relay : Relay  OnSwitchValue=100  OffSwitchValue=70  OnOutputValue=[0 1 -1]  OffOutputValue=[1 0 1]
  Scope : Scope  NumInputPorts=2
  Scope1 : Scope  NumInputPorts=5
  Series RLC Branch1 : spsSeriesRLCBranchLib/Series RLC Branch  LConnTagsString=__new0  RConnTagsString=__new0  BranchType=L  Resistance=1  Inductance=1e-3  SetiL0=off  InitialCurrent=0  Capacitance=1e-6  Setx0=off  InitialVoltage=0  Measurements=None
  Switch : Switch  Criteria=u2 > Threshold
  Voltage Measurement : spsVoltageMeasurementLib/Voltage Measurement  PhasorSimulation=off  OutputType=Complex  PSBequivalent=0
  Vin + : PMIOPort  Side=Left
  Vin - : PMIOPort  Port=2  Side=Left
  Vout + : PMIOPort  Port=3  Side=Right
  Vout - : PMIOPort  Port=4  Side=Right
  State : Outport
  wires:
  Demux/2 -> Mosfet1/1, Scope1/4  "T2"
  Demux/3 -> State/1, Scope1/5  "STATE"
  Demux/1 -> Mosfet3/1, Scope1/3  "T1"
  Voltage Measurement/1 -> Scope/1  "VOLTAGE"
  Current Measurement/1 -> Scope/2  "CURRENT"
  ACTIVATION/1 -> Switch/2
  SOC %/1 -> Scope1/1, Relay/1  "SOC"
  Relay/1 -> Switch/1
  Constant/1 -> Scope1/2, Switch/3
  Switch/1 -> Demux/1
  connections:
  Mosfet3/LConn1 -- Voltage Measurement/LConn1 -- Vout +/RConn1
  Vin -/RConn1 -- Vout -/RConn1 -- Voltage Measurement/LConn2 -- Mosfet1/RConn1
  Mosfet3/RConn1 -- Mosfet1/LConn1 -- Series RLC Branch1/RConn1
  Vin +/RConn1 -- Current Measurement/LConn1
  Series RLC Branch1/LConn1 -- Current Measurement/RConn1

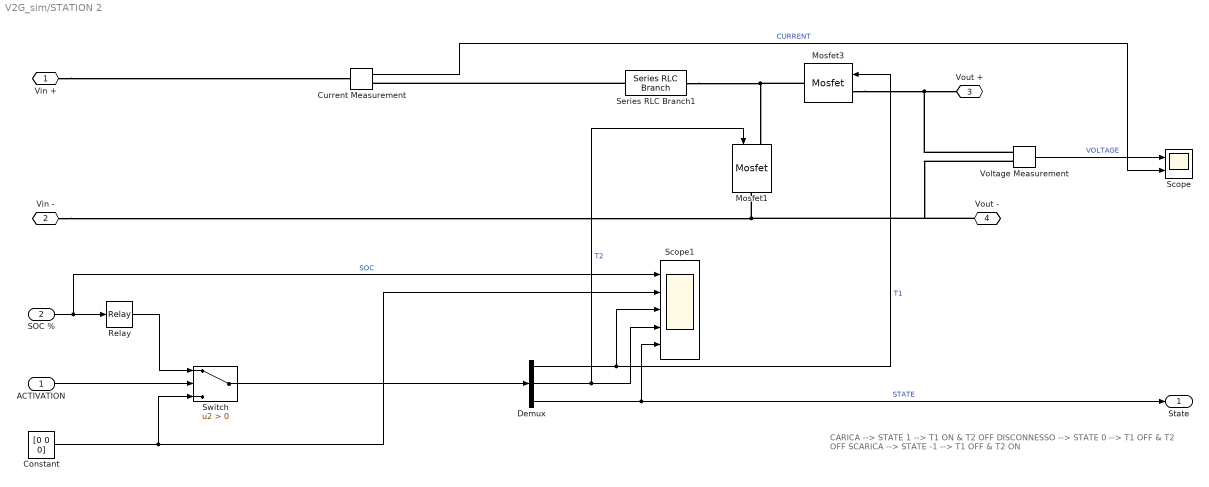
== system V2G_sim/STATION 2 ==
  note: CARICA --> STATE 1 --> T1 ON & T2 OFF
      | DISCONNESSO --> STATE 0 --> T1 OFF & T2 OFF
      | SCARICA --> STATE -1 --> T1 OFF & T2 ON
  ACTIVATION : Inport
  SOC % : Inport  Port=2
  Constant : Constant  Value=[0 0 0]
  Current Measurement : spsCurrentMeasurementLib/Current Measurement  PhasorSimulation=off  OutputType=Complex  PSBequivalent=0
  Demux : Demux  Outputs=3
  Mosfet1 : spsMosfetLib/Mosfet  Ron=0.1  Lon=0  Rd=0.01  Vfd=0  IC=0  Rs=1e5  Cs=inf  Measurements=off
  Mosfet3 : spsMosfetLib/Mosfet  Ron=0.1  Lon=0  Rd=0.01  Vfd=0  IC=0  Rs=1e5  Cs=inf  Measurements=off
  Relay : Relay  OnSwitchValue=100  OffSwitchValue=70  OnOutputValue=[0 1 -1]  OffOutputValue=[1 0 1]
  Scope : Scope  NumInputPorts=2
  Scope1 : Scope  NumInputPorts=5
  Series RLC Branch1 : spsSeriesRLCBranchLib/Series RLC Branch  LConnTagsString=__new0  RConnTagsString=__new0  BranchType=L  Resistance=1  Inductance=1e-3  SetiL0=off  InitialCurrent=0  Capacitance=1e-6  Setx0=off  InitialVoltage=0  Measurements=None
  Switch : Switch  Criteria=u2 > Threshold
  Voltage Measurement : spsVoltageMeasurementLib/Voltage Measurement  PhasorSimulation=off  OutputType=Complex  PSBequivalent=0
  Vin + : PMIOPort  Side=Left
  Vin - : PMIOPort  Port=2  Side=Left
  Vout + : PMIOPort  Port=3  Side=Right
  Vout - : PMIOPort  Port=4  Side=Right
  State : Outport
  wires:
  Demux/2 -> Scope1/4, Mosfet1/1  "T2"
  Demux/3 -> State/1, Scope1/5  "STATE"
  Demux/1 -> Mosfet3/1, Scope1/3  "T1"
  Voltage Measurement/1 -> Scope/1  "VOLTAGE"
  Current Measurement/1 -> Scope/2  "CURRENT"
  ACTIVATION/1 -> Switch/2
  SOC %/1 -> Scope1/1, Relay/1  "SOC"
  Relay/1 -> Switch/1
  Constant/1 -> Scope1/2, Switch/3
  Switch/1 -> Demux/1
  connections:
  Mosfet3/LConn1 -- Vout +/RConn1 -- Voltage Measurement/LConn1
  Vin -/RConn1 -- Mosfet1/RConn1 -- Vout -/RConn1 -- Voltage Measurement/LConn2
  Mosfet3/RConn1 -- Series RLC Branch1/RConn1 -- Mosfet1/LConn1
  Vin +/RConn1 -- Current Measurement/LConn1
  Series RLC Branch1/LConn1 -- Current Measurement/RConn1

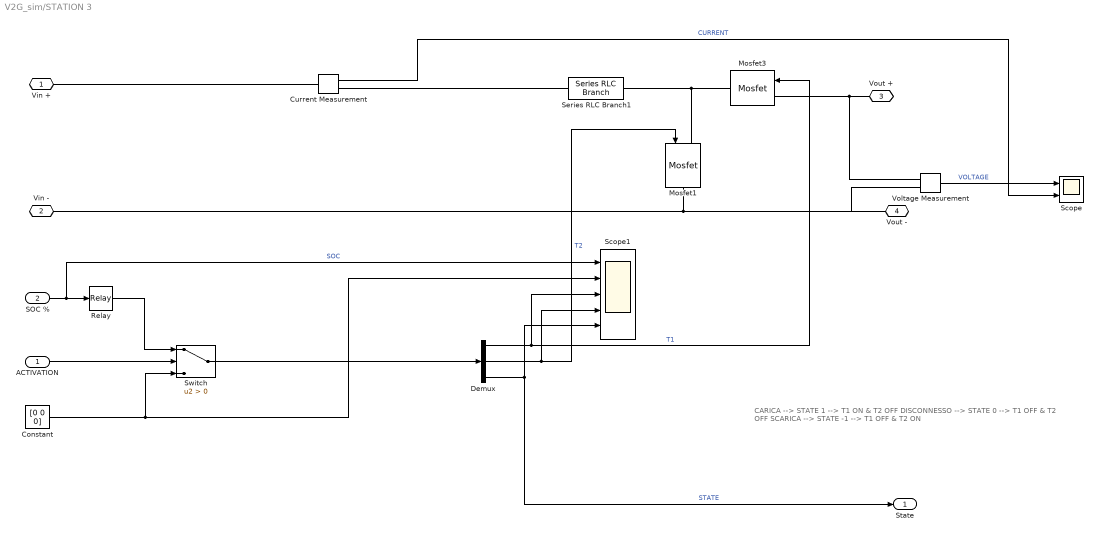
== system V2G_sim/STATION 3 ==
  note: CARICA --> STATE 1 --> T1 ON & T2 OFF
      | DISCONNESSO --> STATE 0 --> T1 OFF & T2 OFF
      | SCARICA --> STATE -1 --> T1 OFF & T2 ON
  ACTIVATION : Inport
  SOC % : Inport  Port=2
  Constant : Constant  Value=[0 0 0]  VectorParams1D=off
  Current Measurement : spsCurrentMeasurementLib/Current Measurement  PhasorSimulation=off  OutputType=Complex  PSBequivalent=0
  Demux : Demux  Outputs=3
  Mosfet1 : spsMosfetLib/Mosfet  Ron=0.1  Lon=0  Rd=0.01  Vfd=0  IC=0  Rs=1e5  Cs=inf  Measurements=off
  Mosfet3 : spsMosfetLib/Mosfet  Ron=0.1  Lon=0  Rd=0.01  Vfd=0  IC=0  Rs=1e5  Cs=inf  Measurements=off
  Relay : Relay  OnSwitchValue=100  OffSwitchValue=70  OnOutputValue=[0 1 -1]  OffOutputValue=[1 0 1]
  Scope : Scope  NumInputPorts=2
  Scope1 : Scope  NumInputPorts=5
  Series RLC Branch1 : spsSeriesRLCBranchLib/Series RLC Branch  LConnTagsString=__new0  RConnTagsString=__new0  BranchType=L  Resistance=1  Inductance=1e-3  SetiL0=off  InitialCurrent=0  Capacitance=1e-6  Setx0=off  InitialVoltage=0  Measurements=None
  Switch : Switch  Criteria=u2 > Threshold
  Voltage Measurement : spsVoltageMeasurementLib/Voltage Measurement  PhasorSimulation=off  OutputType=Complex  PSBequivalent=0
  Vin + : PMIOPort  Side=Left
  Vin - : PMIOPort  Port=2  Side=Left
  Vout + : PMIOPort  Port=3  Side=Right
  Vout - : PMIOPort  Port=4  Side=Right
  State : Outport
  wires:
  Demux/2 -> Mosfet1/1, Scope1/4  "T2"
  Demux/3 -> State/1, Scope1/5  "STATE"
  Demux/1 -> Mosfet3/1, Scope1/3  "T1"
  Voltage Measurement/1 -> Scope/1  "VOLTAGE"
  Current Measurement/1 -> Scope/2  "CURRENT"
  ACTIVATION/1 -> Switch/2
  SOC %/1 -> Scope1/1, Relay/1  "SOC"
  Relay/1 -> Switch/1
  Constant/1 -> Scope1/2, Switch/3
  Switch/1 -> Demux/1
  connections:
  Mosfet3/LConn1 -- Voltage Measurement/LConn1 -- Vout +/RConn1
  Vin -/RConn1 -- Mosfet1/RConn1 -- Vout -/RConn1 -- Voltage Measurement/LConn2
  Mosfet3/RConn1 -- Series RLC Branch1/RConn1 -- Mosfet1/LConn1
  Vin +/RConn1 -- Current Measurement/LConn1
  Series RLC Branch1/LConn1 -- Current Measurement/RConn1

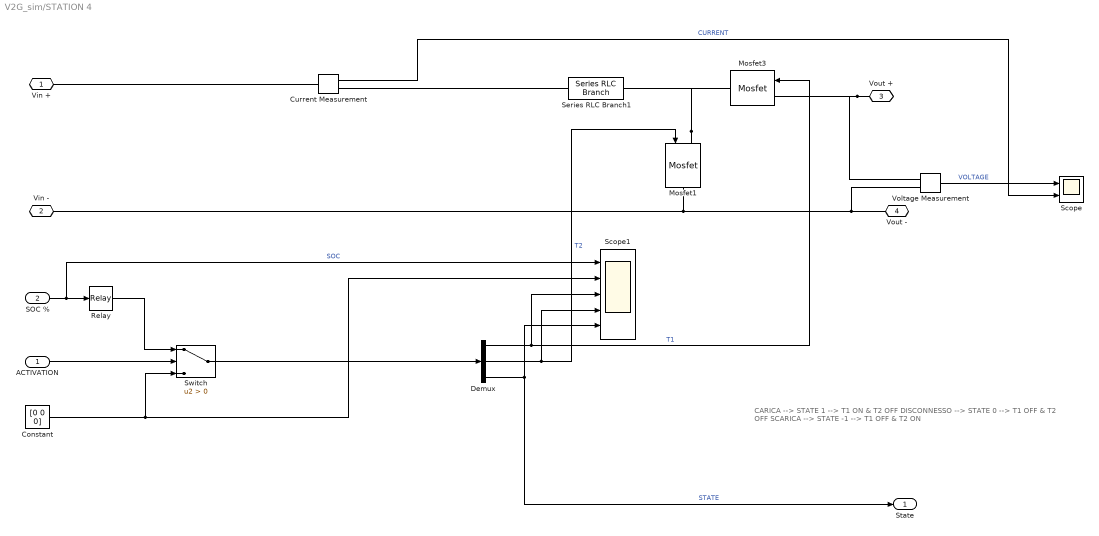
== system V2G_sim/STATION 4 ==
  note: CARICA --> STATE 1 --> T1 ON & T2 OFF
      | DISCONNESSO --> STATE 0 --> T1 OFF & T2 OFF
      | SCARICA --> STATE -1 --> T1 OFF & T2 ON
  ACTIVATION : Inport
  SOC % : Inport  Port=2
  Constant : Constant  Value=[0 0 0]  VectorParams1D=off
  Current Measurement : spsCurrentMeasurementLib/Current Measurement  PhasorSimulation=off  OutputType=Complex  PSBequivalent=0
  Demux : Demux  Outputs=3
  Mosfet1 : spsMosfetLib/Mosfet  Ron=0.1  Lon=0  Rd=0.01  Vfd=0  IC=0  Rs=1e5  Cs=inf  Measurements=off
  Mosfet3 : spsMosfetLib/Mosfet  Ron=0.1  Lon=0  Rd=0.01  Vfd=0  IC=0  Rs=1e5  Cs=inf  Measurements=off
  Relay : Relay  OnSwitchValue=98  OffSwitchValue=70  OnOutputValue=[0 1 -1]  OffOutputValue=[1 0 1]
  Scope : Scope  NumInputPorts=2
  Scope1 : Scope  NumInputPorts=5
  Series RLC Branch1 : spsSeriesRLCBranchLib/Series RLC Branch  LConnTagsString=__new0  RConnTagsString=__new0  BranchType=L  Resistance=1  Inductance=1e-3  SetiL0=off  InitialCurrent=0  Capacitance=1e-6  Setx0=off  InitialVoltage=0  Measurements=None
  Switch : Switch  Criteria=u2 > Threshold
  Voltage Measurement : spsVoltageMeasurementLib/Voltage Measurement  PhasorSimulation=off  OutputType=Complex  PSBequivalent=0
  Vin + : PMIOPort  Side=Left
  Vin - : PMIOPort  Port=2  Side=Left
  Vout + : PMIOPort  Port=3  Side=Right
  Vout - : PMIOPort  Port=4  Side=Right
  State : Outport
  wires:
  Switch/1 -> Demux/1
  Constant/1 -> Switch/3, Scope1/2
  Relay/1 -> Switch/1
  SOC %/1 -> Relay/1, Scope1/1  "SOC"
  ACTIVATION/1 -> Switch/2
  Current Measurement/1 -> Scope/2  "CURRENT"
  Voltage Measurement/1 -> Scope/1  "VOLTAGE"
  Demux/1 -> Scope1/3, Mosfet3/1  "T1"
  Demux/3 -> Scope1/5, State/1  "STATE"
  Demux/2 -> Scope1/4, Mosfet1/1  "T2"
  connections:
  Series RLC Branch1/LConn1 -- Current Measurement/RConn1
  Vin +/RConn1 -- Current Measurement/LConn1
  Mosfet1/LConn1 -- Series RLC Branch1/RConn1 -- Mosfet3/RConn1
  Voltage Measurement/LConn2 -- Vout -/RConn1 -- Mosfet1/RConn1 -- Vin -/RConn1
  Vout +/RConn1 -- Voltage Measurement/LConn1 -- Mosfet3/LConn1

== system V2G_sim/MEASUREMENT 1/Switch Case Action Subsystem ==
  In1 : Inport
  Action Port : ActionPort  PropagateVarSize=During execution  ActionPortLabel=if(u1 > 0)
  CURR_Carica : Outport  OutputWhenDisabled=reset  InitialOutput=0
  wires:
  In1/1 -> CURR_Carica/1

== system V2G_sim/MEASUREMENT 1/Switch Case Action Subsystem1 ==
  In1 : Inport
  Action Port : ActionPort  ActionPortLabel=else
  CURR_Scarica : Outport  OutputWhenDisabled=reset  InitialOutput=0
  wires:
  In1/1 -> CURR_Scarica/1

== system V2G_sim/MEASUREMENT 2/Switch Case Action Subsystem ==
  In1 : Inport
  Action Port : ActionPort  ActionPortLabel=if(u1 > 0)
  CORR_Carica : Outport  OutputWhenDisabled=reset  InitialOutput=0
  wires:
  In1/1 -> CORR_Carica/1

== system V2G_sim/MEASUREMENT 2/Switch Case Action Subsystem1 ==
  In1 : Inport
  Action Port : ActionPort  ActionPortLabel=else
  CORR_Scarica : Outport  OutputWhenDisabled=reset  InitialOutput=0
  wires:
  In1/1 -> CORR_Scarica/1

== system V2G_sim/MEASUREMENT 3 BATTERY/Switch Case Action Subsystem ==
  In1 : Inport
  Action Port : ActionPort  ActionPortLabel=if(u1 > 0)
  CURR_Carica : Outport  OutputWhenDisabled=reset  InitialOutput=0
  wires:
  In1/1 -> CURR_Carica/1

== system V2G_sim/MEASUREMENT 3 BATTERY/Switch Case Action Subsystem1 ==
  In1 : Inport
  Action Port : ActionPort  ActionPortLabel=else
  CURR_Scarica : Outport  OutputWhenDisabled=reset  InitialOutput=0
  wires:
  In1/1 -> CURR_Scarica/1

== system V2G_sim/MEASUREMENT 3 SUPERCAP/Switch Case Action Subsystem ==
  In1 : Inport
  Action Port : ActionPort  ActionPortLabel=if(u1 > 0)
  CORR_Carica : Outport  OutputWhenDisabled=reset  InitialOutput=0
  wires:
  In1/1 -> CORR_Carica/1

== system V2G_sim/MEASUREMENT 3 SUPERCAP/Switch Case Action Subsystem1 ==
  In1 : Inport
  Action Port : ActionPort  ActionPortLabel=else
  CORR_Scarica : Outport  OutputWhenDisabled=reset  InitialOutput=0
  wires:
  In1/1 -> CORR_Scarica/1
